simulink model "Ejercicio_7"  (Simulink 9.2)
settings: Solver=VariableStepAuto  StartTime=0.0  StopTime=10.0  RelTol=1e-3
settings Model: Creator=hathaway  LastModifiedBy=hathaway
settings DataIOCC: LimitDataPoints=off  SaveFormat=Dataset  SignalLoggingSaveFormat=Dataset
settings OptimizationCC: LifeSpan=auto
settings DebuggingCC: UnderspecifiedInitializationDetection=Simplified  MergeDetectMultiDrivingBlocksExec=error  FcnCallInpInsideContextMsg=error  StateNameClashWarn=none  SFUnexpectedBacktrackingDiag=error  SFNoUnconditionalDefaultTransitionDiag=error  SFExecutionAtInitializationDiag=warning
settings HardwareCC: ProdBitPerPointer=64  ProdBitPerSizeT=64  ProdBitPerPtrDiffT=64  ProdLargestAtomicFloat=Float  ProdIntDivRoundTo=Zero  ProdEndianess=LittleEndian  ProdWordSize=64  ProdHWDeviceType=Intel->x86-64 (Windows64)
settings ModelReferenceCC: PropagateSignalLabelsOutOfModel=on
settings SFSimCC: SimUseLocalCustomCode=on
settings RTWCC: RTWUseLocalCustomCode=on
settings CodeAppCC: StateflowObjectComments=off
settings GRTTargetCC: TargetLangStandard=C99 (ISO)  GeneratePreprocessorConditionals=Use local settings  CombineOutputUpdateFcns=on  GRTInterface=off
settings ConfigComp: CovMetricSettings=dwe  CovHtmlReporting=off  CovSaveCumulativeToWorkspaceVar=off  CovSaveSingleToWorkspaceVar=off  CovExternalEMLEnable=on

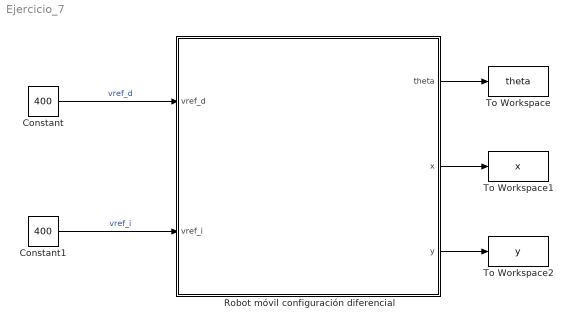
== system Ejercicio_7 ==
  Constant : Constant  Value=400  OutDataTypeStr=double
  Constant1 : Constant  Value=400  OutDataTypeStr=double
  Robot móvil configuración diferencial : Subsystem
  To Workspace : ToWorkspace  VariableName=theta  SaveFormat=Timeseries  SampleTime=-1
  To Workspace1 : ToWorkspace  VariableName=x  SaveFormat=Timeseries  SampleTime=-1
  To Workspace2 : ToWorkspace  VariableName=y  SaveFormat=Timeseries  SampleTime=-1
  wires:
  Constant/1 -> Robot móvil configuración diferencial/1(vref_d)  "vref_d"
  Constant1/1 -> Robot móvil configuración diferencial/2(vref_i)  "vref_i"
  Robot móvil configuración diferencial/1(theta) -> To Workspace/1
  Robot móvil configuración diferencial/2(x) -> To Workspace1/1
  Robot móvil configuración diferencial/3(y) -> To Workspace2/1

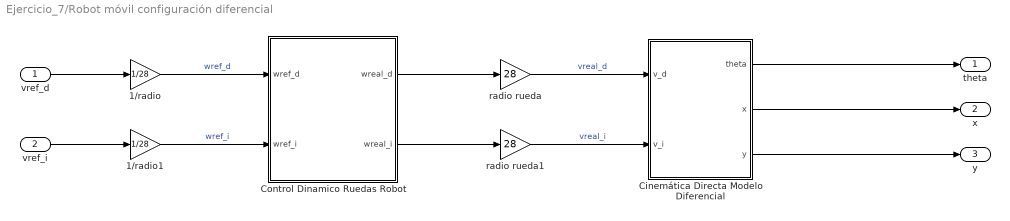
== system Ejercicio_7/Robot móvil configuración diferencial ==
  vref_d : Inport
  vref_i : Inport  Port=2
  1/radio : Gain  Gain=1/28
  1/radio1 : Gain  Gain=1/28
  Cinemática Directa Modelo Diferencial : Subsystem
  Control Dinamico Ruedas Robot : Subsystem
  radio rueda : Gain  Gain=28
  radio rueda1 : Gain  Gain=28
  theta : Outport
  x : Outport  Port=2
  y : Outport  Port=3
  wires:
  1/radio1/1 -> Control Dinamico Ruedas Robot/2(wref_i)  "wref_i"
  vref_i/1 -> 1/radio1/1
  Cinemática Directa Modelo Diferencial/3(y) -> y/1
  1/radio/1 -> Control Dinamico Ruedas Robot/1(wref_d)  "wref_d"
  Control Dinamico Ruedas Robot/1(wreal_d) -> radio rueda/1
  vref_d/1 -> 1/radio/1
  radio rueda/1 -> Cinemática Directa Modelo Diferencial/1(v_d)  "vreal_d"
  radio rueda1/1 -> Cinemática Directa Modelo Diferencial/2(v_i)  "vreal_i"
  Control Dinamico Ruedas Robot/2(wreal_i) -> radio rueda1/1
  Cinemática Directa Modelo Diferencial/2(x) -> x/1
  Cinemática Directa Modelo Diferencial/1(theta) -> theta/1

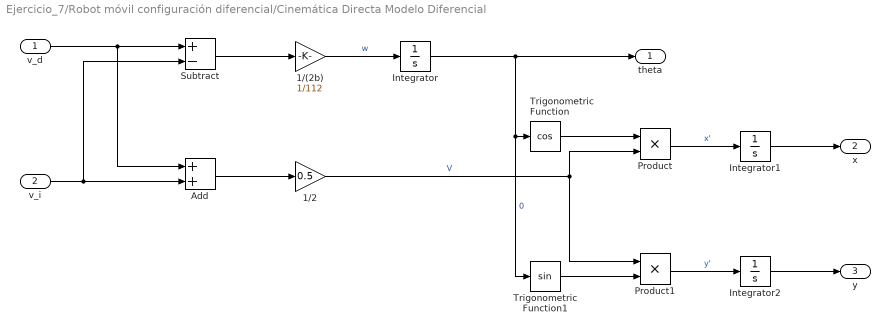
== system Ejercicio_7/Robot móvil configuración diferencial/Cinemática Directa Modelo Diferencial ==
  v_d : Inport
  v_i : Inport  Port=2
  1/(2b) : Gain  Gain=1/112
  1/2 : Gain  Gain=0.5
  Add : Sum
  Integrator : Integrator
  Integrator1 : Integrator
  Integrator2 : Integrator
  Product : Product
  Product1 : Product
  Subtract : Sum  Inputs=+-
  Trigonometric Function : Trigonometry  Operator=cos
  Trigonometric Function1 : Trigonometry
  theta : Outport
  x : Outport  Port=2
  y : Outport  Port=3
  wires:
  Add/1 -> 1/2/1
  v_i/1 -> Subtract/2, Add/2
  v_d/1 -> Add/1, Subtract/1
  Integrator2/1 -> y/1
  Integrator/1 -> theta/1, Trigonometric Function1/1, Trigonometric Function/1  "0"
  Subtract/1 -> 1/(2b)/1
  Product1/1 -> Integrator2/1  "y'"
  1/(2b)/1 -> Integrator/1  "w"
  1/2/1 -> Product/2, Product1/1  "V"
  Trigonometric Function1/1 -> Product1/2
  Trigonometric Function/1 -> Product/1
  Product/1 -> Integrator1/1  "x'"
  Integrator1/1 -> x/1

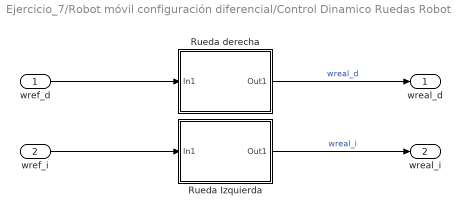
== system Ejercicio_7/Robot móvil configuración diferencial/Control Dinamico Ruedas Robot ==
  wref_d : Inport
  wref_i : Inport  Port=2
  Rueda Izquierda : Subsystem  mask{k=0.2, tau=0.09, kp=3}
      mask prompts: k "Valor ganancia del motor:"; tau "Valor cte tiempo motor:"; kp "Valor ganancia regulador P:"
  Rueda derecha : Subsystem  mask{k=0.2, tau=0.09, kp=3}
      mask prompts: k "Valor ganancia del motor:"; tau "Valor cte tiempo motor:"; kp "Valor ganancia regulador P:"
  wreal_d : Outport
  wreal_i : Outport  Port=2
  wires:
  wref_i/1 -> Rueda Izquierda/1(In1)
  Rueda derecha/1(Out1) -> wreal_d/1  "wreal_d"
  Rueda Izquierda/1(Out1) -> wreal_i/1  "wreal_i"
  wref_d/1 -> Rueda derecha/1(In1)

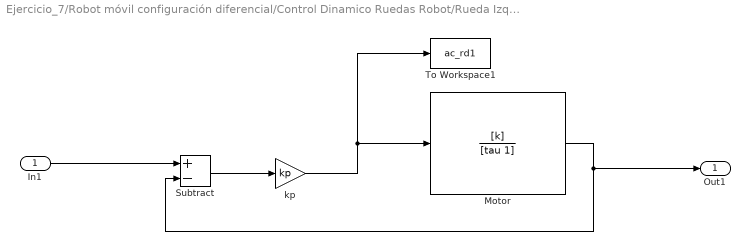
== system Ejercicio_7/Robot móvil configuración diferencial/Control Dinamico Ruedas Robot/Rueda Izquierda ==
  In1 : Inport
  Motor : TransferFcn  Numerator=[k]  Denominator=[tau 1]
  Subtract : Sum  Inputs=+-
  To Workspace1 : ToWorkspace  VariableName=ac_rd1  SaveFormat=Timeseries  SampleTime=-1
  kp : Gain  Gain=kp
  Out1 : Outport
  wires:
  Motor/1 -> Out1/1, Subtract/2
  kp/1 -> To Workspace1/1, Motor/1
  Subtract/1 -> kp/1
  In1/1 -> Subtract/1

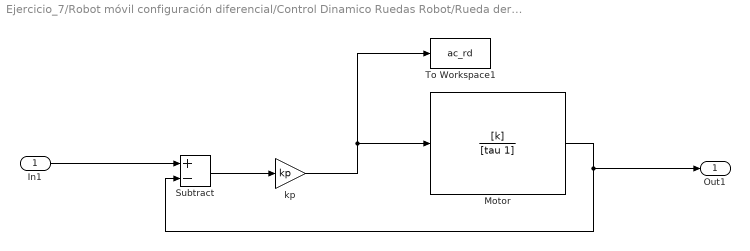
== system Ejercicio_7/Robot móvil configuración diferencial/Control Dinamico Ruedas Robot/Rueda derecha ==
  In1 : Inport
  Motor : TransferFcn  Numerator=[k]  Denominator=[tau 1]
  Subtract : Sum  Inputs=+-
  To Workspace1 : ToWorkspace  VariableName=ac_rd  SaveFormat=Timeseries  SampleTime=-1
  kp : Gain  Gain=kp
  Out1 : Outport
  wires:
  In1/1 -> Subtract/1
  Subtract/1 -> kp/1
  kp/1 -> Motor/1, To Workspace1/1
  Motor/1 -> Subtract/2, Out1/1
